simulink model "impedanceControl_new_wbi_ID"  (Simulink 8.3)
settings: Solver=FixedStepDiscrete  StartTime=0.0  StopTime=Inf  FixedStep=Ts  RelTol=1e-3
InitFcn:
  | init_new_wbi_ID;
libraries: WBCLibrary x9
settings Model: Creator=daniele  LastModifiedBy=jorhabib
settings DebuggingCC: UnderspecifiedInitializationDetection=Simplified  MultiTaskDSMMsg=warning  MultiTaskCondExecSysMsg=none  StateNameClashWarn=none  StrictBusMsg=ErrorOnBusTreatedAsVector
settings RTWCC: IncludeERTFirstTime=on
settings GRTTargetCC: CombineOutputUpdateFcns=on  GRTInterface=off

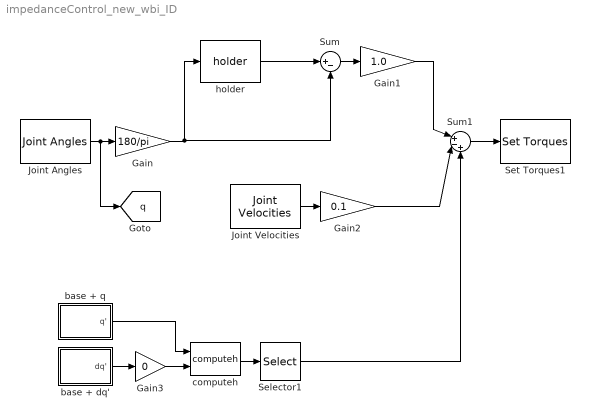
== system impedanceControl_new_wbi_ID ==
  Gain : Gain  Gain=180/pi
  Gain1 : Gain  Gain=1.0
  Gain2 : Gain  Gain=0.1
  Gain3 : Gain  Gain=0
  Joint Angles : WBCLibrary/wholeBodyStates/Joint Angles  robotName=robotName  localName=localName
  Joint Velocities : WBCLibrary/wholeBodyStates/Joint Velocities  robotName=robotName  localName=localName
  Selector1 : Selector  InputPortWidth=8  Indices=[7:8]
  Set Torques1 : WBCLibrary/wholeBodyActuators/Set Torques  val=6  robotName=robotName  localName=localName
  Sum : Sum  Inputs=|+-
  Sum1 : Sum  Inputs=|+-+
  base + dq' : Subsystem
  base + q : Subsystem
  computeh : WBCLibrary/wholeBodyModel/Dynamics/computeh  val=7  robotname=robotName  localname=localName
  "holder " : WBCLibrary/Utilities/holder 
  tag scope: q=global
  wires:
  Joint Angles/1 -> [q], Gain/1
  Gain/1 -> Sum/2, "holder "/1
  "holder "/1 -> Sum/1
  Sum/1 -> Gain1/1
  Gain1/1 -> Sum1/1
  Joint Velocities/1 -> Gain2/1
  Gain2/1 -> Sum1/2
  Sum1/1 -> Set Torques1/1
  base + q/1(q') -> computeh/1
  Gain3/1 -> computeh/2
  base + dq'/1(dq') -> Gain3/1
  computeh/1 -> Selector1/1
  Selector1/1 -> Sum1/3

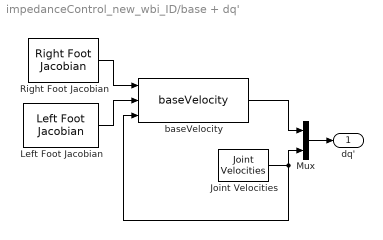
== system impedanceControl_new_wbi_ID/base + dq' ==
  Joint Velocities : WBCLibrary/wholeBodyStates/Joint Velocities  robotName=robotName  localName=localName
  Left Foot Jacobian : WBCLibrary/wholeBodyModel/Jacobians/Left Foot Jacobian  robotName=robotName  localName=localName
  Mux : Mux  Inputs=2
  Right Foot Jacobian : WBCLibrary/wholeBodyModel/Jacobians/Right Foot Jacobian  robotName=robotName  localName=localName
  baseVelocity : WBCLibrary/Utilities/baseVelocity
  dq' : Outport
  wires:
  Left Foot Jacobian/1 -> baseVelocity/2
  Right Foot Jacobian/1 -> baseVelocity/1
  baseVelocity/1 -> Mux/1
  Joint Velocities/1 -> baseVelocity/3, Mux/2
  Mux/1 -> dq'/1

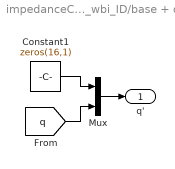
== system impedanceControl_new_wbi_ID/base + q ==
  Constant1 : Constant  Value=zeros(16,1)
  Mux : Mux  Inputs=2
  q' : Outport
  wires:
  Mux/1 -> q'/1
  [q] -> Mux/2
  Constant1/1 -> Mux/1
